simulink model "sim_Observer_based_OKID_closed_loop"  (R2014b)
settings: Solver=ode45  StartTime=0.0  StopTime=10.0  RelTol=1e-3
values from neighbouring files (symbols this model uses):
  A = zp2ss(2, P ,8)    [OKID_closed_loop.m]
  B = H    [OKID_closed_loop.m]    (also in OKID_fun_WT02_6.m = Btemp(:, 1:r))
  C = [-4.268707812 5.80698373674 2.29894982459 -1.81972727507 -0.693726564507 -1.15322974081 0.496155860115 0.368426779263]    [OKIDData.mat]
  Kd = place(G,H,Pd)    [OKID_closed_loop.m]
  Ts = 1800    [OKIDData.mat]    (also in OKID_closed_loop.m = 0.005)
undefined symbols (not defined in the file or in its folder): C_ok, F_ok, G_ok, H_ok
settings Model: Creator=123  LastModifiedBy=123

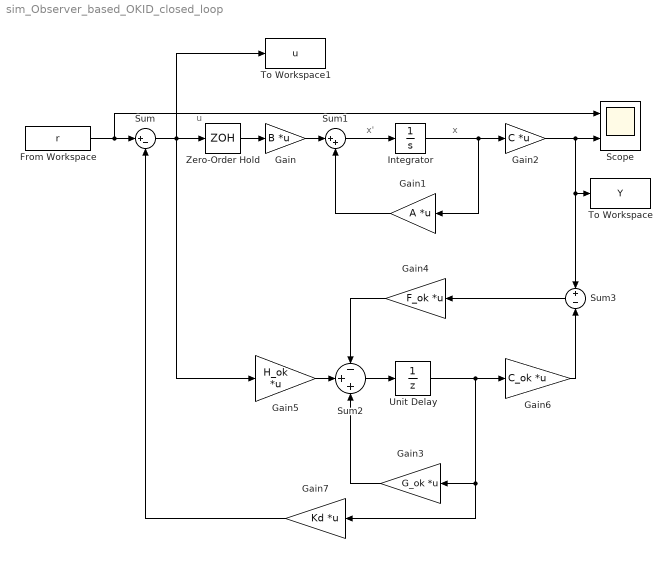
== system sim_Observer_based_OKID_closed_loop ==
  note: u
  note: x'
  note: x
  From Workspace : FromWorkspace  VariableName=r  SampleTime=0
  Gain : Gain  Gain=B  Multiplication=Matrix(K*u)
  Gain1 : Gain  Gain=A  Multiplication=Matrix(K*u)
  Gain2 : Gain  Gain=C  Multiplication=Matrix(K*u)
  Gain3 : Gain  Gain=G_ok  Multiplication=Matrix(K*u)
  Gain4 : Gain  Gain=F_ok  Multiplication=Matrix(K*u)
  Gain5 : Gain  Gain=H_ok  Multiplication=Matrix(K*u)
  Gain6 : Gain  Gain=C_ok  Multiplication=Matrix(K*u)
  Gain7 : Gain  Gain=Kd  Multiplication=Matrix(K*u)
  Integrator : Integrator  InitialCondition=1
  Scope : Scope  NumInputPorts=2
      settings: YMin=-5~-5  YMax=5~5
  Sum : Sum  Inputs=|+-
  Sum1 : Sum  Inputs=|++
  Sum2 : Sum  Inputs=-++
  Sum3 : Sum  Inputs=+|-
  To Workspace : ToWorkspace  VariableName=Y  SampleTime=-1
  To Workspace1 : ToWorkspace  VariableName=u  SampleTime=-1
  Unit Delay : UnitDelay  InitialCondition=1  SampleTime=Ts
  Zero-Order Hold : ZeroOrderHold  SampleTime=Ts
  wires:
  Integrator/1 -> Gain1/1, Gain2/1
  Sum/1 -> Gain5/1, Zero-Order Hold/1, To Workspace1/1
  From Workspace/1 -> Sum/1, Scope/1
  Sum1/1 -> Integrator/1
  Gain/1 -> Sum1/1
  Gain1/1 -> Sum1/2
  Gain2/1 -> To Workspace/1, Sum3/1, Scope/2
  Zero-Order Hold/1 -> Gain/1
  Unit Delay/1 -> Gain7/1, Gain3/1, Gain6/1
  Gain5/1 -> Sum2/2
  Sum2/1 -> Unit Delay/1
  Gain3/1 -> Sum2/3
  Gain6/1 -> Sum3/2
  Sum3/1 -> Gain4/1
  Gain4/1 -> Sum2/1
  Gain7/1 -> Sum/2
